simulink model "RT_Klausur_2010"  (R2013a)
settings: Solver=ode45  StartTime=0.0  StopTime=10.0  RelTol=1e-3
settings Model: Creator=mainster  LastModifiedBy=mainster

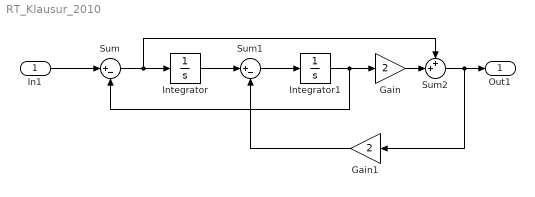
== system RT_Klausur_2010 ==
  In1 : Inport
  Gain : Gain  Gain=2
  Gain1 : Gain  Gain=2
  Integrator : Integrator
  Integrator1 : Integrator
  Sum : Sum  Inputs=|+-
  Sum1 : Sum  Inputs=|+-
  Sum2 : Sum  Inputs=++|
  Out1 : Outport
  wires:
  In1/1 -> Sum/1
  Sum/1 -> Sum2/1, Integrator/1
  Integrator/1 -> Sum1/1
  Sum1/1 -> Integrator1/1
  Integrator1/1 -> Sum/2, Gain/1
  Gain/1 -> Sum2/2
  Sum2/1 -> Gain1/1, Out1/1
  Gain1/1 -> Sum1/2
